simulink model "spacecraft_attitude_model"  (R2024b)
settings: Solver=ode4  StartTime=t0  StopTime=tf  FixedStep=0.1  RelTol=1e-3
values from neighbouring files (symbols this model uses):
  a = (((T/(2*pi))^2*mu_earth)^(1/3))    (= 7069867.85099)    [main_spacecraft_attitude_dynamics.m]
  A_body1 = surface(1)    [main_spacecraft_attitude_dynamics.m]
  A_body2 = surface(2)    [main_spacecraft_attitude_dynamics.m]
  A_body3 = surface(3)    [main_spacecraft_attitude_dynamics.m]
  A_body4 = surface(4)    [main_spacecraft_attitude_dynamics.m]
  A_body5 = surface(5)    [main_spacecraft_attitude_dynamics.m]
  A_body6 = surface(6)    [main_spacecraft_attitude_dynamics.m]
  A_panel1 = surface(7)    [main_spacecraft_attitude_dynamics.m]
  A_panel2 = surface(8)    [main_spacecraft_attitude_dynamics.m]
  A_panel3 = surface(9)    [main_spacecraft_attitude_dynamics.m]
  A_panel4 = surface(10)    [main_spacecraft_attitude_dynamics.m]
  alpha = [alpha1,alpha2,alpha3]    [main_spacecraft_attitude_dynamics.m]
  Ap = pinv(Ar)    [main_spacecraft_attitude_dynamics.m]
  Ar = Ar./norm(Ar)    [main_spacecraft_attitude_dynamics.m]
  AtmosphereModel = struct()    [AtmosphereData.m]    (also in main_spacecraft_attitude_dynamics.m)
  CD = 2.6    [main_spacecraft_attitude_dynamics.m]
  D_max = 50    [main_spacecraft_attitude_dynamics.m]
  Detumbling_time = 5000    [main_spacecraft_attitude_dynamics.m]
  e = 0.001    [main_spacecraft_attitude_dynamics.m]
  FOV = 128 * pi/180    (= 2.23402144255)    [main_spacecraft_attitude_dynamics.m]
  g1_0 = DGRF2020(1).g_nm    [main_spacecraft_attitude_dynamics.m]
  g1_1 = DGRF2020(2).g_nm    [main_spacecraft_attitude_dynamics.m]
  H = 700    [main_spacecraft_attitude_dynamics.m]
  h0 = 0    [main_spacecraft_attitude_dynamics.m]
  h1_1 = DGRF2020(2).h_nm    [main_spacecraft_attitude_dynamics.m]
  i = deg2rad(98.18)    [main_spacecraft_attitude_dynamics.m]
  Ir = 0.1    [main_spacecraft_attitude_dynamics.m]
  J = EXTRACTED_DATA.I_total    [main_spacecraft_attitude_dynamics.m]
  j_B = [0.01, 0.05, 0.01]'    [main_spacecraft_attitude_dynamics.m]
  k1 = max(max(kd_slew))    [main_spacecraft_attitude_dynamics.m]
  k2 = max(max(kp_slew))    [main_spacecraft_attitude_dynamics.m]
  Kw = max(max(kp_detumbling))    [main_spacecraft_attitude_dynamics.m]
  n = sqrt((G*M_E)/(r_earth^3))    [main_spacecraft_attitude_dynamics.m]
  N_B1 = N_B(1, :)'    [main_spacecraft_attitude_dynamics.m]
  N_B2 = N_B(2, :)'    [main_spacecraft_attitude_dynamics.m]
  N_B3 = N_B(3, :)'    [main_spacecraft_attitude_dynamics.m]
  N_B4 = N_B(4, :)'    [main_spacecraft_attitude_dynamics.m]
  N_B5 = N_B(5, :)'    [main_spacecraft_attitude_dynamics.m]
  N_B6 = N_B(6, :)'    [main_spacecraft_attitude_dynamics.m]
  N_P1 = N_B(7, :)'    [main_spacecraft_attitude_dynamics.m]
  N_P2 = N_B(8, :)'    [main_spacecraft_attitude_dynamics.m]
  N_P3 = N_B(9, :)'    [main_spacecraft_attitude_dynamics.m]
  N_P4 = N_B(10, :)'    [main_spacecraft_attitude_dynamics.m]
  n_S = (2*pi)/T_S    (= 1.99238499086e-07)    [main_spacecraft_attitude_dynamics.m]
  om = deg2rad(0)    [main_spacecraft_attitude_dynamics.m]
  P = Fe/c    (= 4.52980041279e-06)    [main_spacecraft_attitude_dynamics.m]
  pd_body1 = rho_D(1)    [main_spacecraft_attitude_dynamics.m]
  pd_body2 = rho_D(2)    [main_spacecraft_attitude_dynamics.m]
  pd_body3 = rho_D(3)    [main_spacecraft_attitude_dynamics.m]
  pd_body4 = rho_D(4)    [main_spacecraft_attitude_dynamics.m]
  pd_body5 = rho_D(5)    [main_spacecraft_attitude_dynamics.m]
  pd_body6 = rho_D(6)    [main_spacecraft_attitude_dynamics.m]
  pd_panel1 = rho_D(7)    [main_spacecraft_attitude_dynamics.m]
  pd_panel2 = rho_D(8)    [main_spacecraft_attitude_dynamics.m]
  pd_panel3 = rho_D(9)    [main_spacecraft_attitude_dynamics.m]
  pd_panel4 = rho_D(10)    [main_spacecraft_attitude_dynamics.m]
  ps_body1 = rho_S(1)    [main_spacecraft_attitude_dynamics.m]
  ps_body2 = rho_S(2)    [main_spacecraft_attitude_dynamics.m]
  ps_body3 = rho_S(3)    [main_spacecraft_attitude_dynamics.m]
  ps_body4 = rho_S(4)    [main_spacecraft_attitude_dynamics.m]
  ps_body5 = rho_S(5)    [main_spacecraft_attitude_dynamics.m]
  ps_body6 = rho_S(6)    [main_spacecraft_attitude_dynamics.m]
  ps_panel1 = rho_S(7)    [main_spacecraft_attitude_dynamics.m]
  ps_panel2 = rho_S(8)    [main_spacecraft_attitude_dynamics.m]
  ps_panel3 = rho_S(9)    [main_spacecraft_attitude_dynamics.m]
  ps_panel4 = rho_S(10)    [main_spacecraft_attitude_dynamics.m]
  q0 = [q1_0 q2_0 q3_0 q4_0]    [main_spacecraft_attitude_dynamics.m]
  r_earth = (R_earth + H)*10^3    (= 7078136.3)    [main_spacecraft_attitude_dynamics.m]
  R_earth = 6378.1363    [main_spacecraft_attitude_dynamics.m]
  r_f1 = r_F(1, :)'    [main_spacecraft_attitude_dynamics.m]
  r_f10 = r_F(10, :)'    [main_spacecraft_attitude_dynamics.m]
  r_f2 = r_F(2, :)'    [main_spacecraft_attitude_dynamics.m]
  r_f3 = r_F(3, :)'    [main_spacecraft_attitude_dynamics.m]
  r_f4 = r_F(4, :)'    [main_spacecraft_attitude_dynamics.m]
  r_f5 = r_F(5, :)'    [main_spacecraft_attitude_dynamics.m]
  r_f6 = r_F(6, :)'    [main_spacecraft_attitude_dynamics.m]
  r_f7 = r_F(7, :)'    [main_spacecraft_attitude_dynamics.m]
  r_f8 = r_F(8, :)'    [main_spacecraft_attitude_dynamics.m]
  r_f9 = r_F(9, :)'    [main_spacecraft_attitude_dynamics.m]
  r_Sun = 149597870    [main_spacecraft_attitude_dynamics.m]
  RAAN = deg2rad(RAAN)    [main_spacecraft_attitude_dynamics.m]
  sigma_b = RRW*(pi/180)*(1/3600)*(1/sqrt(Ts))    [main_spacecraft_attitude_dynamics.m]
  sigma_mag = 10^-6    (= 1e-06)    [main_spacecraft_attitude_dynamics.m]
  sigma_n = ARW*(pi/180)*(1/60)*(1/sqrt(Ts))    [main_spacecraft_attitude_dynamics.m]
  T_coil_max = 50 * 45*10^-6    (= 0.00225)    [main_spacecraft_attitude_dynamics.m]
  th0 = 0    [main_spacecraft_attitude_dynamics.m]
  v0 = [0 0 0]    [main_spacecraft_attitude_dynamics.m]
  variance_Ss = (a_sun)^2    (= 3.24)    [main_spacecraft_attitude_dynamics.m]
  w_0 = [-3, 3, 3]'    [main_spacecraft_attitude_dynamics.m]
  w_E = (2*pi)/(24*60*60)    (= 7.27220521664e-05)    [main_spacecraft_attitude_dynamics.m]
  w_LN = [0 0 0]'    [main_spacecraft_attitude_dynamics.m]
undefined symbols (not defined in the file or in its folder): A_Ss_orienation
libraries: matrix_library x38, slpidlib x2, aerolibutil x1, vrlib x1
(part 3 of 4)

== system spacecraft_attitude_model/Slew & Pointing/Slew and Pointing/Subsystem ==
  q_referance : Inport
  q_measured : Inport  Port=2
  Demux : Demux
  Gain : Gain  Gain=[0 0 0 -1; 0 0 1 0; 0 -1 0 0; 1 0 0 0];
  Gain1 : Gain  Gain=[0 1 0 0; -1 0 0 0; 0 0 0 -1; 0 0 1 0];
  Gain2 : Gain  Gain=[0 0 -1 0; 0 0 0 -1; 1 0 0 0; 0 1 0 0];
  Gain3 : Gain  Gain=[1 0 0 0; 0 1 0 0; 0 0 1 0; 0 0 0 1];
  MatrixMultiply : Product  Multiplication=Matrix(*)
  Sum : Sum  Inputs=++++
  q_error : Outport
  wires:
  q_referance/1 -> Demux/1
  Demux/1 -> Gain/1
  Demux/3 -> Gain1/1
  Demux/2 -> Gain2/1
  Demux/4 -> Gain3/1
  Gain/1 -> Sum/1
  Gain2/1 -> Sum/2
  Gain1/1 -> Sum/3
  Gain3/1 -> Sum/4
  Sum/1 -> MatrixMultiply/1
  q_measured/1 -> MatrixMultiply/2
  MatrixMultiply/1 -> q_error/1

== system spacecraft_attitude_model/Slew & Pointing/Slew and Pointing/Subsystem1 ==
  A_LN : Inport
  Clock : Clock
  Clock1 : Clock
  If : If  NumInputs=4  IfExpression=u1>0 & u1<1  ElseIfExpressions=u2>0 & u2<1, u3>0 & u3<1, u4>0 & u4<1  ShowElse=off
  If Action Subsystem : Subsystem  TreatAsAtomicUnit=on
  If Action Subsystem1 : Subsystem  TreatAsAtomicUnit=on
  If Action Subsystem2 : Subsystem  TreatAsAtomicUnit=on
  If Action Subsystem3 : Subsystem  TreatAsAtomicUnit=on
  If Action Subsystem4 : Subsystem  TreatAsAtomicUnit=on
  If Action Subsystem5 : Subsystem  TreatAsAtomicUnit=on
  If1 : If  IfExpression=u1==0
  Merge : Merge  Inputs=4
  Ortonormalization : Subsystem
  Scope : Scope
  Subsystem : Subsystem
  Subsystem1 : Subsystem
  Subsystem2 : Subsystem
  Subsystem3 : Subsystem
  Switch : Switch  Criteria=u2 ~= 0  SaturateOnIntegerOverflow=off  InputSameDT=off
  q : Outport
  wires:
  A_LN/1 -> Ortonormalization/1(A_LN)
  If/1 -> If Action Subsystem/Action
  If Action Subsystem/1(quaternion_4) -> Merge/1
  Merge/1 -> If Action Subsystem5/1(In1), If Action Subsystem1/1(In1)
  Subsystem/1(q4) -> If Action Subsystem/1(q4), If/1
  Subsystem1/1(q1) -> If Action Subsystem2/1(q1), If/2
  Subsystem2/1(q2) -> If/3, If Action Subsystem3/1(q2)
  Subsystem3/1(q3) -> If Action Subsystem4/1(q3), If/4
  If/2 -> If Action Subsystem2/Action
  If/3 -> If Action Subsystem3/Action
  If/4 -> If Action Subsystem4/Action
  If Action Subsystem2/1(quaternion_1) -> Merge/2
  If Action Subsystem3/1(quaternion_2) -> Merge/3
  If Action Subsystem4/1(quaternion_3) -> Merge/4
  Ortonormalization/1(Out1) -> If Action Subsystem3/2(A_BN), If Action Subsystem4/2("A_BN "), If Action Subsystem/2("A_BN "), If Action Subsystem2/2("A_BN "), Subsystem3/1(A_BN), Subsystem/1(A_BN), Subsystem1/1(A_BN), Subsystem2/1(A_BN)
  Clock/1 -> If1/1
  If1/1 -> If Action Subsystem1/Action
  If1/2 -> If Action Subsystem5/Action
  If Action Subsystem1/1(q) -> Switch/3
  If Action Subsystem5/1(q) -> Switch/1
  Switch/1 -> Scope/1, q/1
  Clock1/1 -> Switch/2

== system spacecraft_attitude_model/Slew & Pointing/Slew and Pointing/Subsystem2 ==
  q : Inport
  Clock : Clock
  Clock1 : Clock
  If Action Subsystem1 : Subsystem  TreatAsAtomicUnit=on
  If Action Subsystem5 : Subsystem  TreatAsAtomicUnit=on
  If1 : If  IfExpression=u1==0
  Scope1 : Scope
  Switch : Switch  Criteria=u2 ~= 0  SaturateOnIntegerOverflow=off  InputSameDT=off
  q_referance : Outport
  wires:
  If Action Subsystem1/1(q) -> Switch/3
  If Action Subsystem5/1(q_) -> Switch/1
  If1/1 -> If Action Subsystem1/Action
  Clock/1 -> If1/1
  Switch/1 -> q_referance/1, Scope1/1
  Clock1/1 -> Switch/2
  If1/2 -> If Action Subsystem5/Action
  q/1 -> If Action Subsystem1/1(Input), If Action Subsystem5/1(In1)

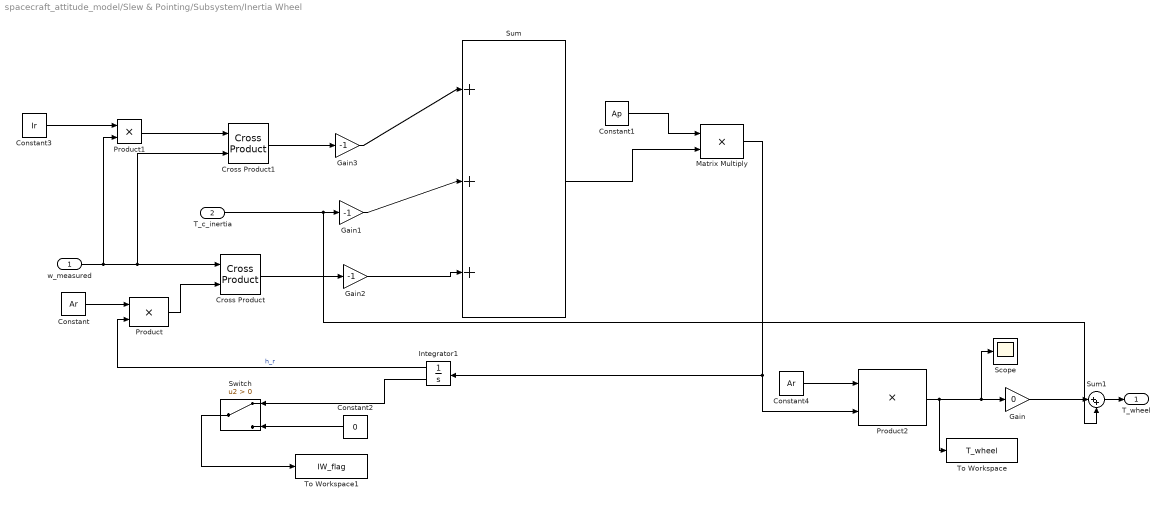
== system spacecraft_attitude_model/Slew & Pointing/Subsystem/Inertia Wheel ==
  w_measured : Inport
  T_c_inertia : Inport  Port=2
  Constant : Constant  Value=Ar
  Constant1 : Constant  Value=Ap
  Constant2 : Constant  Value=0
  Constant3 : Constant  Value=Ir
  Constant4 : Constant  Value=Ar
  Cross Product : matrix_library/Cross Product
  Cross Product1 : matrix_library/Cross Product
  Gain : Gain  Gain=0
  Gain1 : Gain  Gain=-1
  Gain2 : Gain  Gain=-1
  Gain3 : Gain  Gain=-1
  Integrator1 : Integrator  InitialCondition=h0  LimitOutput=on  UpperSaturationLimit=0.005  LowerSaturationLimit=-0.005  ShowSaturationPort=on
  Matrix Multiply : Product
  Product : Product
  Product1 : Product
  Product2 : Product
  Scope : Scope
  Sum : Sum  Inputs=|+++
  Sum1 : Sum  Inputs=|++
  Switch : Switch  Criteria=u2 > Threshold  SaturateOnIntegerOverflow=off  InputSameDT=off
  To Workspace : ToWorkspace  VariableName=T_wheel  SampleTime=-1
  To Workspace1 : ToWorkspace  VariableName=IW_flag  SampleTime=-1
  T_wheel : Outport
  wires:
  Product/1 -> Cross Product/2
  Cross Product/1 -> Gain2/1
  w_measured/1 -> Product1/2, Cross Product1/2, Cross Product/1
  Gain2/1 -> Sum/3
  Constant1/1 -> Matrix Multiply/1
  Gain3/1 -> Sum/1
  Matrix Multiply/1 -> Product2/2, Integrator1/1
  Constant3/1 -> Product1/1
  Integrator1/1 -> Product/2  "h_r"
  Integrator1/2 -> Switch/1
  Constant2/1 -> Switch/3
  Constant/1 -> Product/1
  Product2/1 -> To Workspace/1, Scope/1, Gain/1
  Gain1/1 -> Sum/2
  Switch/1 -> To Workspace1/1
  Product1/1 -> Cross Product1/1
  Cross Product1/1 -> Gain3/1
  Constant4/1 -> Product2/1
  T_c_inertia/1 -> Sum1/2, Gain1/1
  Sum/1 -> Matrix Multiply/2
  Gain/1 -> Sum1/1
  Sum1/1 -> T_wheel/1

== system spacecraft_attitude_model/Slew & Pointing/Subsystem/Magnetic coils ==
  T_Control : Inport
  b_measured : Inport  Port=2
  Demux : Demux  Outputs=3
  Demux1 : Demux  Outputs=3
  Gain : Gain
  Gain1 : Gain
  Gain2 : Gain
  Norm1 : Subsystem
      settings: PortSchema="{\"entries\":[{\"content\":{\"sides\":[{\"content\":{},\"type\":\"ConnectorPlacement.EquallySpacedRectSide\",\"uuid\":\"c8e6b557-1f56-4290-9ece-bfc368650609\"},{\"content\":{\"connectorIds\":[\"Out1\"],\"side\":\"RIGHT\"},\"type\":\"ConnectorPlacement.EquallySpacedRectSide\",\"uuid\":\"77fa52b5-00ea-4466-8814-b89029d0f61f\"},{\"content\":{\"connectorIds\":[\"In1\"],\"side\":\"TOP\"},\"type\":\"ConnectorPlacement.EquallySpacedRectSide\",\"uuid\":\"5a1e965d-5eef-4834-963c-decfdd4da2be\"},{\"content\":{\"side\":\"BOTTOM\"},\"type\":\"ConnectorPlacement.EquallySpacedRectSide\",\"uuid\":\"d0b05173-3d81-4b7c-baba-8d47e4810e0f\"}]},\"type\":\"ConnectorPlacement.EquallySpacedConnector\",\"uuid\":\"bc13670f-664f-40fc-b4f3-9fab538d09d1\"}],\"packageUris\":[\"http://schema.mathworks.com/mf0/Connector/R2020b\"],\"version\":\"1.0\"}"
  Scope2 : Scope
  Square1 : Math  Operator=square
  Subsystem : Subsystem
  Subsystem1 : Subsystem
  Subsystem2 : Subsystem
  Vector Concatenate : Concatenate  NumInputs=3
  T_coils : Outport
  wires:
  Square1/1 -> Subsystem/3(b_norm^2), Subsystem1/3(b_norm^2), Subsystem2/3(b_norm^2)
  Demux1/2 -> Subsystem1/2(b_y)
  Demux/1 -> Gain/1
  Demux1/1 -> Subsystem/2(b_x)
  Gain1/1 -> Subsystem1/1(T_y)
  Gain/1 -> Subsystem/1(T_x)
  Gain2/1 -> Subsystem2/1(T_z)
  Demux1/3 -> Subsystem2/2(b_z)
  Demux/3 -> Gain2/1
  b_measured/1 -> Norm1/1(b), Demux1/1
  Norm1/1(b_norm) -> Square1/1  "b_norm"
  Demux/2 -> Gain1/1
  Vector Concatenate/1 -> T_coils/1, Scope2/1
  T_Control/1 -> Demux/1
  Subsystem2/1(T_coil_z) -> Vector Concatenate/3
  Subsystem1/1(T_coil_y) -> Vector Concatenate/2
  Subsystem/1(T_coil_x) -> Vector Concatenate/1

== system spacecraft_attitude_model/Sun Sensor /Alpha Beta1/Subsystem ==
  In1 : Inport
  Atan1 : Trigonometry  Operator=atan2
  Atan2 : Trigonometry  Operator=atan2
  Demux : Demux  Outputs=3
  Out1 : Outport
  Out2 : Outport  Port=2
  wires:
  Demux/3 -> Atan2/2, Atan1/2  "Sz"
  Atan1/1 -> Out2/1
  Demux/1 -> Atan2/1  "Sx"
  In1/1 -> Demux/1
  Demux/2 -> Atan1/1  "Sy"
  Atan2/1 -> Out1/1

== system spacecraft_attitude_model/Sun Sensor /Alpha Beta1/Subsystem1 ==
  In1 : Inport
  Atan1 : Trigonometry  Operator=atan2
  Atan2 : Trigonometry  Operator=atan2
  Demux : Demux  Outputs=3
  Out1 : Outport
  Out2 : Outport  Port=2
  wires:
  Demux/3 -> Atan2/2, Atan1/2  "Sz"
  Atan1/1 -> Out2/1
  Demux/1 -> Atan2/1  "Sx"
  In1/1 -> Demux/1
  Demux/2 -> Atan1/1  "Sy"
  Atan2/1 -> Out1/1

== system spacecraft_attitude_model/Sun Sensor /Alpha Beta1/Subsystem2 ==
  In1 : Inport
  Atan1 : Trigonometry  Operator=atan2
  Atan2 : Trigonometry  Operator=atan2
  Demux : Demux  Outputs=3
  Out1 : Outport
  Out2 : Outport  Port=2
  wires:
  Demux/3 -> Atan2/2, Atan1/2  "Sz"
  Atan1/1 -> Out2/1
  Demux/1 -> Atan2/1  "Sx"
  In1/1 -> Demux/1
  Demux/2 -> Atan1/1  "Sy"
  Atan2/1 -> Out1/1

== system spacecraft_attitude_model/Sun Sensor /Alpha Beta1/Subsystem3 ==
  In1 : Inport
  Atan1 : Trigonometry  Operator=atan2
  Atan2 : Trigonometry  Operator=atan2
  Demux : Demux  Outputs=3
  Out1 : Outport
  Out2 : Outport  Port=2
  wires:
  Demux/3 -> Atan2/2, Atan1/2  "Sz"
  Atan1/1 -> Out2/1
  Demux/1 -> Atan2/1  "Sx"
  In1/1 -> Demux/1
  Demux/2 -> Atan1/1  "Sy"
  Atan2/1 -> Out1/1

== system spacecraft_attitude_model/Sun Sensor /Alpha Beta1/Subsystem4 ==
  In1 : Inport
  Atan1 : Trigonometry  Operator=atan2
  Atan2 : Trigonometry  Operator=atan2
  Demux : Demux  Outputs=3
  Out1 : Outport
  Out2 : Outport  Port=2
  wires:
  Demux/3 -> Atan2/2, Atan1/2  "Sz"
  Atan1/1 -> Out2/1
  Demux/1 -> Atan2/1  "Sx"
  In1/1 -> Demux/1
  Demux/2 -> Atan1/1  "Sy"
  Atan2/1 -> Out1/1

== system spacecraft_attitude_model/Sun Sensor /Alpha Beta1/Subsystem5 ==
  In1 : Inport
  Atan1 : Trigonometry  Operator=atan2
  Atan2 : Trigonometry  Operator=atan2
  Demux : Demux  Outputs=3
  Out1 : Outport
  Out2 : Outport  Port=2
  wires:
  Demux/3 -> Atan2/2, Atan1/2  "Sz"
  Atan1/1 -> Out2/1
  Demux/1 -> Atan2/1  "Sx"
  In1/1 -> Demux/1
  Demux/2 -> Atan1/1  "Sy"
  Atan2/1 -> Out1/1

== system spacecraft_attitude_model/Detumbling/Subsystem4/Magnetic coils/Norm1 ==
  b : Inport
  Demux : Demux  Outputs=3
  Sqrt : Sqrt
  Square : Math  Operator=square
  Square1 : Math  Operator=square
  Square2 : Math  Operator=square
  Sum : Sum  Inputs=|+++
  b_norm : Outport
  wires:
  Demux/3 -> Square2/1
  b/1 -> Demux/1
  Demux/1 -> Square/1
  Demux/2 -> Square1/1
  Square/1 -> Sum/1
  Square1/1 -> Sum/2
  Square2/1 -> Sum/3
  Sum/1 -> Sqrt/1
  Sqrt/1 -> b_norm/1

== system spacecraft_attitude_model/Detumbling/Subsystem4/Magnetic coils/Subsystem ==
  T_x : Inport
  b_x : Inport  Port=2
  b_norm^2 : Inport  Port=3
  Divide2 : Product  Inputs=*/
  Product : Product
  Product1 : Product
  Saturation2 : Saturate  UpperLimit=T_coil_max  LowerLimit=-T_coil_max
  Saturation3 : Saturate  UpperLimit=D_max  LowerLimit=-D_max
  Scope2 : Scope
  Scope3 : Scope
  T_coil_x : Outport
  wires:
  Saturation3/1 -> Product1/1
  Divide2/1 -> Scope3/1, Saturation3/1
  Product/1 -> Divide2/1
  Product1/1 -> Saturation2/1  "T_coils_x"
  b_norm^2/1 -> Divide2/2
  b_x/1 -> Product1/2, Product/2
  T_x/1 -> Product/1
  Saturation2/1 -> Scope2/1, T_coil_x/1

== system spacecraft_attitude_model/Detumbling/Subsystem4/Magnetic coils/Subsystem1 ==
  T_y : Inport
  b_y : Inport  Port=2
  b_norm^2 : Inport  Port=3
  Divide2 : Product  Inputs=*/
  Product : Product
  Product1 : Product
  Saturation2 : Saturate  UpperLimit=T_coil_max  LowerLimit=-T_coil_max
  Saturation3 : Saturate  UpperLimit=D_max  LowerLimit=-D_max
  Scope2 : Scope
  Scope3 : Scope
  T_coil_y : Outport
  wires:
  Saturation3/1 -> Product1/1
  Divide2/1 -> Scope3/1, Saturation3/1
  Product/1 -> Divide2/1
  Product1/1 -> Saturation2/1
  b_norm^2/1 -> Divide2/2
  b_y/1 -> Product1/2, Product/2
  T_y/1 -> Product/1
  Saturation2/1 -> Scope2/1, T_coil_y/1

== system spacecraft_attitude_model/Detumbling/Subsystem4/Magnetic coils/Subsystem2 ==
  T_z : Inport
  b_z : Inport  Port=2
  b_norm^2 : Inport  Port=3
  Divide2 : Product  Inputs=*/
  Product : Product
  Product1 : Product
  Saturation2 : Saturate  UpperLimit=T_coil_max  LowerLimit=-T_coil_max
  Saturation3 : Saturate  UpperLimit=D_max  LowerLimit=-D_max
  Scope2 : Scope
  Scope3 : Scope
  T_coil_z : Outport
  wires:
  Saturation3/1 -> Product1/1
  Divide2/1 -> Scope3/1, Saturation3/1
  Product/1 -> Divide2/1
  Product1/1 -> Saturation2/1
  b_norm^2/1 -> Divide2/2
  b_z/1 -> Product1/2, Product/2
  T_z/1 -> Product/1
  Saturation2/1 -> Scope2/1, T_coil_z/1

== system spacecraft_attitude_model/Disturbances Torque/Air Drag/A_Cross/A_CROSS1 ==
  v_r_hat : Inport
  A_1 : Constant  Value=A_body1
  Constant : Constant  Value=0
  Dot Product : DotProduct  OutDataTypeStr=Inherit: Inherit via internal rule
  Product : Product
  Switch : Switch  SaturateOnIntegerOverflow=off  InputSameDT=off
  n_s1 : Constant  Value=N_B1
  A_cross1 : Outport
  wires:
  n_s1/1 -> Dot Product/1
  Dot Product/1 -> Product/2, Switch/2
  Switch/1 -> A_cross1/1
  Constant/1 -> Switch/3
  Product/1 -> Switch/1
  A_1/1 -> Product/1
  v_r_hat/1 -> Dot Product/2

== system spacecraft_attitude_model/Disturbances Torque/Air Drag/A_Cross/A_CROSS10 ==
  v_r_hat : Inport
  A_10 : Constant  Value=A_panel4
  Constant : Constant  Value=0
  Dot Product : DotProduct  OutDataTypeStr=Inherit: Inherit via internal rule
  Product : Product
  Switch : Switch  SaturateOnIntegerOverflow=off  InputSameDT=off
  n_s10 : Constant  Value=N_P4
  A_cross10 : Outport
  wires:
  n_s10/1 -> Dot Product/1
  Dot Product/1 -> Product/2, Switch/2
  Switch/1 -> A_cross10/1
  Constant/1 -> Switch/3
  Product/1 -> Switch/1
  A_10/1 -> Product/1
  v_r_hat/1 -> Dot Product/2

== system spacecraft_attitude_model/Disturbances Torque/Air Drag/A_Cross/A_CROSS2 ==
  v_r_hat : Inport
  A_2 : Constant  Value=A_body2
  Constant : Constant  Value=0
  Dot Product : DotProduct  OutDataTypeStr=Inherit: Inherit via internal rule
  Product : Product
  Switch : Switch  SaturateOnIntegerOverflow=off  InputSameDT=off
  n_s2 : Constant  Value=N_B2
  A_cross2 : Outport
  wires:
  n_s2/1 -> Dot Product/1
  Dot Product/1 -> Product/2, Switch/2
  Switch/1 -> A_cross2/1
  Constant/1 -> Switch/3
  Product/1 -> Switch/1
  A_2/1 -> Product/1
  v_r_hat/1 -> Dot Product/2

== system spacecraft_attitude_model/Disturbances Torque/Air Drag/A_Cross/A_CROSS3 ==
  v_r_hat : Inport
  A_3 : Constant  Value=A_body3
  Constant : Constant  Value=0
  Dot Product : DotProduct  OutDataTypeStr=Inherit: Inherit via internal rule
  Product : Product
  Switch : Switch  SaturateOnIntegerOverflow=off  InputSameDT=off
  n_s3 : Constant  Value=N_B3
  A_cross3 : Outport
  wires:
  n_s3/1 -> Dot Product/1
  Dot Product/1 -> Product/2, Switch/2
  Switch/1 -> A_cross3/1
  Constant/1 -> Switch/3
  Product/1 -> Switch/1
  A_3/1 -> Product/1
  v_r_hat/1 -> Dot Product/2

== system spacecraft_attitude_model/Disturbances Torque/Air Drag/A_Cross/A_CROSS4 ==
  v_r_hat : Inport
  A_4 : Constant  Value=A_body4
  Constant : Constant  Value=0
  Dot Product : DotProduct  OutDataTypeStr=Inherit: Inherit via internal rule
  Product : Product
  Switch : Switch  SaturateOnIntegerOverflow=off  InputSameDT=off
  n_s4 : Constant  Value=N_B4
  A_cross4 : Outport
  wires:
  n_s4/1 -> Dot Product/1
  Dot Product/1 -> Product/2, Switch/2
  Switch/1 -> A_cross4/1
  Constant/1 -> Switch/3
  Product/1 -> Switch/1
  A_4/1 -> Product/1
  v_r_hat/1 -> Dot Product/2

== system spacecraft_attitude_model/Disturbances Torque/Air Drag/A_Cross/A_CROSS5 ==
  v_r_hat : Inport
  A_5 : Constant  Value=A_body5
  Constant : Constant  Value=0
  Dot Product : DotProduct  OutDataTypeStr=Inherit: Inherit via internal rule
  Product : Product
  Switch : Switch  SaturateOnIntegerOverflow=off  InputSameDT=off
  n_s5 : Constant  Value=N_B5
  A_cross2 : Outport
  wires:
  n_s5/1 -> Dot Product/1
  Dot Product/1 -> Product/2, Switch/2
  Switch/1 -> A_cross2/1
  Constant/1 -> Switch/3
  Product/1 -> Switch/1
  A_5/1 -> Product/1
  v_r_hat/1 -> Dot Product/2

== system spacecraft_attitude_model/Disturbances Torque/Air Drag/A_Cross/A_CROSS6 ==
  v_r_hat : Inport
  A_6 : Constant  Value=A_body6
  Constant : Constant  Value=0
  Dot Product : DotProduct  OutDataTypeStr=Inherit: Inherit via internal rule
  Product : Product
  Switch : Switch  SaturateOnIntegerOverflow=off  InputSameDT=off
  n_s6 : Constant  Value=N_B6
  A_cross6 : Outport
  wires:
  n_s6/1 -> Dot Product/1
  Dot Product/1 -> Product/2, Switch/2
  Switch/1 -> A_cross6/1
  Constant/1 -> Switch/3
  Product/1 -> Switch/1
  A_6/1 -> Product/1
  v_r_hat/1 -> Dot Product/2

== system spacecraft_attitude_model/Disturbances Torque/Air Drag/A_Cross/A_CROSS7 ==
  v_r_hat : Inport
  A_7 : Constant  Value=A_panel1
  Constant : Constant  Value=0
  Dot Product : DotProduct  OutDataTypeStr=Inherit: Inherit via internal rule
  Product : Product
  Switch : Switch  SaturateOnIntegerOverflow=off  InputSameDT=off
  n_s7 : Constant  Value=N_P1
  A_cross7 : Outport
  wires:
  n_s7/1 -> Dot Product/1
  Dot Product/1 -> Product/2, Switch/2
  Switch/1 -> A_cross7/1
  Constant/1 -> Switch/3
  Product/1 -> Switch/1
  A_7/1 -> Product/1
  v_r_hat/1 -> Dot Product/2

== system spacecraft_attitude_model/Disturbances Torque/Air Drag/A_Cross/A_CROSS8 ==
  v_r_hat : Inport
  A_8 : Constant  Value=A_panel2
  Constant : Constant  Value=0
  Dot Product : DotProduct  OutDataTypeStr=Inherit: Inherit via internal rule
  Product : Product
  Switch : Switch  SaturateOnIntegerOverflow=off  InputSameDT=off
  n_s8 : Constant  Value=N_P2
  A_cross8 : Outport
  wires:
  n_s8/1 -> Dot Product/1
  Dot Product/1 -> Product/2, Switch/2
  Switch/1 -> A_cross8/1
  Constant/1 -> Switch/3
  Product/1 -> Switch/1
  A_8/1 -> Product/1
  v_r_hat/1 -> Dot Product/2

== system spacecraft_attitude_model/Disturbances Torque/Air Drag/A_Cross/A_CROSS9 ==
  v_r_hat : Inport
  A_9 : Constant  Value=A_panel3
  Constant : Constant  Value=0
  Dot Product : DotProduct  OutDataTypeStr=Inherit: Inherit via internal rule
  Product : Product
  Switch : Switch  SaturateOnIntegerOverflow=off  InputSameDT=off
  n_s9 : Constant  Value=N_P3
  A_cross9 : Outport
  wires:
  n_s9/1 -> Dot Product/1
  Dot Product/1 -> Product/2, Switch/2
  Switch/1 -> A_cross9/1
  Constant/1 -> Switch/3
  Product/1 -> Switch/1
  A_9/1 -> Product/1
  v_r_hat/1 -> Dot Product/2

== system spacecraft_attitude_model/Disturbances Torque/Air Drag/Subsystem1/F1 ==
  v_rB^2 : Inport
  v_rB_hat : Inport  Port=2
  A_cross1 : Inport  Port=3
  Constant : Constant  Value=-1/2
  Constant1 : Constant  Value=CD
  Product : Product  Inputs=6
  rho : Constant  Value=AtmosphereModel(H/100).Density_kg_m3/10^6
  Out1 : Outport
  wires:
  rho/1 -> Product/2
  Constant1/1 -> Product/3
  Constant/1 -> Product/1
  v_rB^2/1 -> Product/4
  Product/1 -> Out1/1
  v_rB_hat/1 -> Product/5
  A_cross1/1 -> Product/6

== system spacecraft_attitude_model/Disturbances Torque/Air Drag/Subsystem1/F10 ==
  v_rB^2 : Inport
  v_rB_hat : Inport  Port=2
  A_cross10 : Inport  Port=3
  Constant : Constant  Value=-1/2
  Constant1 : Constant  Value=CD
  Product : Product  Inputs=6
  rho : Constant  Value=AtmosphereModel(H/100).Density_kg_m3/10^6
  Out1 : Outport
  wires:
  rho/1 -> Product/2
  Constant1/1 -> Product/3
  Constant/1 -> Product/1
  v_rB^2/1 -> Product/4
  Product/1 -> Out1/1
  v_rB_hat/1 -> Product/5
  A_cross10/1 -> Product/6

== system spacecraft_attitude_model/Disturbances Torque/Air Drag/Subsystem1/F2 ==
  v_rB^2 : Inport
  v_rB_hat : Inport  Port=2
  A_cross2 : Inport  Port=3
  Constant : Constant  Value=-1/2
  Constant1 : Constant  Value=CD
  Product : Product  Inputs=6
  rho : Constant  Value=AtmosphereModel(H/100).Density_kg_m3/10^6
  Out1 : Outport
  wires:
  rho/1 -> Product/2
  Constant1/1 -> Product/3
  Constant/1 -> Product/1
  v_rB^2/1 -> Product/4
  Product/1 -> Out1/1
  v_rB_hat/1 -> Product/5
  A_cross2/1 -> Product/6

== system spacecraft_attitude_model/Disturbances Torque/Air Drag/Subsystem1/F3 ==
  v_rB^2 : Inport
  v_rB_hat : Inport  Port=2
  A_cross3 : Inport  Port=3
  Constant : Constant  Value=-1/2
  Constant1 : Constant  Value=CD
  Product : Product  Inputs=6
  rho : Constant  Value=AtmosphereModel(H/100).Density_kg_m3/10^6
  Out1 : Outport
  wires:
  rho/1 -> Product/2
  Constant1/1 -> Product/3
  Constant/1 -> Product/1
  v_rB^2/1 -> Product/4
  Product/1 -> Out1/1
  v_rB_hat/1 -> Product/5
  A_cross3/1 -> Product/6

== system spacecraft_attitude_model/Disturbances Torque/Air Drag/Subsystem1/F4 ==
  v_rB^2 : Inport
  v_rB_hat : Inport  Port=2
  A_cross4 : Inport  Port=3
  Constant : Constant  Value=-1/2
  Constant1 : Constant  Value=CD
  Product : Product  Inputs=6
  rho : Constant  Value=AtmosphereModel(H/100).Density_kg_m3/10^6
  Out1 : Outport
  wires:
  rho/1 -> Product/2
  Constant1/1 -> Product/3
  Constant/1 -> Product/1
  v_rB^2/1 -> Product/4
  Product/1 -> Out1/1
  v_rB_hat/1 -> Product/5
  A_cross4/1 -> Product/6

== system spacecraft_attitude_model/Disturbances Torque/Air Drag/Subsystem1/F5 ==
  v_rB^2 : Inport
  v_rB_hat : Inport  Port=2
  A_cross5 : Inport  Port=3
  Constant : Constant  Value=-1/2
  Constant1 : Constant  Value=CD
  Product : Product  Inputs=6
  rho : Constant  Value=AtmosphereModel(H/100).Density_kg_m3/10^6
  Out1 : Outport
  wires:
  rho/1 -> Product/2
  Constant1/1 -> Product/3
  Constant/1 -> Product/1
  v_rB^2/1 -> Product/4
  Product/1 -> Out1/1
  v_rB_hat/1 -> Product/5
  A_cross5/1 -> Product/6

== system spacecraft_attitude_model/Disturbances Torque/Air Drag/Subsystem1/F6 ==
  v_rB^2 : Inport
  v_rB_hat : Inport  Port=2
  A_cross6 : Inport  Port=3
  Constant : Constant  Value=-1/2
  Constant1 : Constant  Value=CD
  Product : Product  Inputs=6
  rho : Constant  Value=AtmosphereModel(H/100).Density_kg_m3/10^6
  Out1 : Outport
  wires:
  rho/1 -> Product/2
  Constant1/1 -> Product/3
  Constant/1 -> Product/1
  v_rB^2/1 -> Product/4
  Product/1 -> Out1/1
  v_rB_hat/1 -> Product/5
  A_cross6/1 -> Product/6

== system spacecraft_attitude_model/Disturbances Torque/Air Drag/Subsystem1/F7 ==
  v_rB^2 : Inport
  v_rB_hat : Inport  Port=2
  A_cross7 : Inport  Port=3
  Constant : Constant  Value=-1/2
  Constant1 : Constant  Value=CD
  Product : Product  Inputs=6
  rho : Constant  Value=AtmosphereModel(H/100).Density_kg_m3/10^6
  Out1 : Outport
  wires:
  rho/1 -> Product/2
  Constant1/1 -> Product/3
  Constant/1 -> Product/1
  v_rB^2/1 -> Product/4
  Product/1 -> Out1/1
  v_rB_hat/1 -> Product/5
  A_cross7/1 -> Product/6

== system spacecraft_attitude_model/Disturbances Torque/Air Drag/Subsystem1/F8 ==
  v_rB^2 : Inport
  v_rB_hat : Inport  Port=2
  A_cross8 : Inport  Port=3
  Constant : Constant  Value=-1/2
  Constant1 : Constant  Value=CD
  Product : Product  Inputs=6
  rho : Constant  Value=AtmosphereModel(H/100).Density_kg_m3/10^6
  Out1 : Outport
  wires:
  rho/1 -> Product/2
  Constant1/1 -> Product/3
  Constant/1 -> Product/1
  v_rB^2/1 -> Product/4
  Product/1 -> Out1/1
  v_rB_hat/1 -> Product/5
  A_cross8/1 -> Product/6

== system spacecraft_attitude_model/Disturbances Torque/Air Drag/Subsystem1/F9 ==
  v_rB^2 : Inport
  v_rB_hat : Inport  Port=2
  A_cross9 : Inport  Port=3
  Constant : Constant  Value=-1/2
  Constant1 : Constant  Value=CD
  Product : Product  Inputs=6
  rho : Constant  Value=AtmosphereModel(H/100).Density_kg_m3/10^6
  Out1 : Outport
  wires:
  rho/1 -> Product/2
  Constant1/1 -> Product/3
  Constant/1 -> Product/1
  v_rB^2/1 -> Product/4
  Product/1 -> Out1/1
  v_rB_hat/1 -> Product/5
  A_cross9/1 -> Product/6

== system spacecraft_attitude_model/Disturbances Torque/Gravity Gradient/Gravity Gradient/c ==
  A_BL : Inport
  Constant : Constant  Value=0
  Constant1 : Constant
  Matrix Multiply : Product  Multiplication=Matrix(*)
  Mux : Mux  Inputs=3
  c : Outport
  wires:
  Constant1/1 -> Mux/1
  Constant/1 -> Mux/3, Mux/2
  A_BL/1 -> Matrix Multiply/1
  Mux/1 -> Matrix Multiply/2
  Matrix Multiply/1 -> c/1

== system spacecraft_attitude_model/Envoirment/Model/Magnetic Field/H0 ==
  Constant : Constant  Value=(g1_0)^2
  Constant1 : Constant  Value=(g1_1)^2
  Constant2 : Constant  Value=(h1_1)^2
  Scope : Scope
  Sqrt : Sqrt
  Sum : Sum  Inputs=|+++
  To Workspace : ToWorkspace  VariableName=H0  SampleTime=-1
  H_0 : Outport
  wires:
  Constant2/1 -> Sum/3
  Sum/1 -> Sqrt/1
  Sqrt/1 -> To Workspace/1, Scope/1, H_0/1
  Constant/1 -> Sum/1
  Constant1/1 -> Sum/2

== system spacecraft_attitude_model/Envoirment/Model/Magnetic Field/b_Ned ==
  m : Inport
  H_0 : Inport  Port=2
  r_N : Inport  Port=3
  Constant : Constant  Value=3
  Constant1 : Constant  Value=(r_earth)^3
  Divide : Product  Inputs=*/
  Divide1 : Product  Inputs=*/
  Dot Product : DotProduct  OutDataTypeStr=Inherit: Inherit via internal rule
  Gain : Gain  Gain=3
  Norm : Subsystem
  Power : Math  Operator=pow
  Product : Product
  Product2 : Product
  Product3 : Product
  Scope : Scope
  Scope1 : Scope
  Scope2 : Scope
  Sum : Sum  Inputs=|+-
  b_N : Outport
  wires:
  H_0/1 -> Product/1
  m/1 -> Dot Product/1, Sum/2
  Dot Product/1 -> Product2/1  "m * r"
  r_N/1 -> Divide1/1, Norm/1(In1)
  Norm/1(Out1) -> Scope1/1, Power/1, Divide1/2  "r_norm"
  Divide1/1 -> Scope2/1, Dot Product/2, Product2/2  "r_versor"
  Constant/1 -> Power/2
  Product/1 -> Product3/2
  Product3/1 -> Divide/1
  Power/1 -> Divide/2
  Divide/1 -> Scope/1, b_N/1
  Sum/1 -> Product3/1  "3(m*r)r - m"
  Product2/1 -> Gain/1  "(m*r)r"
  Gain/1 -> Sum/1
  Constant1/1 -> Product/2

== system spacecraft_attitude_model/Envoirment/Model/Magnetic Field/m ==
  11.5 deg : Constant  Value=deg2rad(11.5)
  Clock : Clock
  Constant : Constant  Value=w_E
  Cos : Trigonometry  Operator=cos
  Cos1 : Trigonometry  Operator=cos
  Product : Product
  Product1 : Product
  Product2 : Product
  Scope : Scope
  Sin : Trigonometry
  Sin1 : Trigonometry
  Vector Concatenate : Concatenate  NumInputs=3
  m : Outport
  wires:
  Product2/1 -> Vector Concatenate/2
  Clock/1 -> Product/1
  11.5 deg/1 -> Sin/1, Cos/1
  Sin/1 -> Product2/1, Product1/1
  Cos1/1 -> Product1/2
  Cos/1 -> Vector Concatenate/3
  Sin1/1 -> Product2/2
  Constant/1 -> Product/2
  Product1/1 -> Vector Concatenate/1
  Vector Concatenate/1 -> Scope/1, m/1
  Product/1 -> Sin1/1, Cos1/1

== system spacecraft_attitude_model/Envoirment/Two_Body_Keplerian_Dynamics/Subsystem/rN ==
  r : Inport
  Theta : Inport  Port=2
  Constant : Constant  Value=deg2rad(98.18)
  Cos1 : Trigonometry  Operator=cos
  Cos3 : Trigonometry  Operator=cos
  Product{,1..4} (5 alike) : Product
  Sin : Trigonometry
  Sin1 : Trigonometry
  Vector Concatenate : Concatenate  NumInputs=3
  r_N : Outport
  wires:
  Theta/1 -> Cos3/1, Sin1/1
  Constant/1 -> Sin/1, Cos1/1
  Product4/1 -> Vector Concatenate/3  "r*sin(th)*sin(i)"
  Product/1 -> Vector Concatenate/1  "r*cos(th)"
  Product2/1 -> Vector Concatenate/2  "r*sin(th)*cos(i)"
  r/1 -> Product4/1, Product2/1, Product/1  "r"
  Sin1/1 -> Product3/1, Product1/1
  Product1/1 -> Product2/2
  Cos3/1 -> Product/2
  Sin/1 -> Product3/2
  Product3/1 -> Product4/2
  Vector Concatenate/1 -> r_N/1
  Cos1/1 -> Product1/2

== system spacecraft_attitude_model/Kinematics/quaternions to DCM/q2A_DCM/Creation of q vector skew Matrix ==
  q : Inport
  Constant : Constant  Value=[1 0 0]
  Constant1 : Constant  Value=[0 1 0]  VectorParams1D=off
  Constant2 : Constant  Value=[0 0 1]  VectorParams1D=off
  Cross Product : matrix_library/Cross Product
  Cross Product1 : matrix_library/Cross Product
  Cross Product2 : matrix_library/Cross Product
  Matrix Concatenate : Concatenate  NumInputs=3  Mode=Multidimensional array
  To Workspace1 : ToWorkspace  VariableName=q_skew  SampleTime=-1
  Transpose : matrix_library/Transpose
  "[q]^" : Outport
  wires:
  q/1 -> Cross Product/1, Cross Product1/1, Cross Product2/1
  Constant2/1 -> Cross Product2/2
  Cross Product1/1 -> Matrix Concatenate/2  "Line 2"
  Cross Product2/1 -> Matrix Concatenate/3  "Line 3"
  Cross Product/1 -> Matrix Concatenate/1  "Line 1"
  Matrix Concatenate/1 -> Transpose/1  "skew"
  Constant1/1 -> Cross Product1/2
  Constant/1 -> Cross Product/2
  Transpose/1 -> To Workspace1/1, "[q]^"/1

== system spacecraft_attitude_model/Slew & Pointing/Slew and Pointing/Subsystem1/If Action Subsystem ==
  q4 : Inport
  "A_BN " : Inport  Port=2
  Action Port : ActionPort  ActionPortLabel=if(u1>0 & u1<1)
  Divide : Product  Inputs=*/
  Divide1 : Product  Inputs=*/
  Divide2 : Product  Inputs=*/
  Gain1 : Gain  Gain=1/4
  Gain2 : Gain  Gain=1/4
  Gain3 : Gain  Gain=1/4
  Mux : Mux
  Selector : Selector  NumberOfDimensions=2  InputPortWidth=3  IndexOptions=Index vector (dialog),Index vector (dialog)  Indices=2,3  OutputSizes=1,1
  Selector1 : Selector  NumberOfDimensions=2  InputPortWidth=3  IndexOptions=Index vector (dialog),Index vector (dialog)  Indices=3,2  OutputSizes=1,1
  Selector2 : Selector  NumberOfDimensions=2  InputPortWidth=3  IndexOptions=Index vector (dialog),Index vector (dialog)  Indices=3,1  OutputSizes=1,1
  Selector3 : Selector  NumberOfDimensions=2  InputPortWidth=3  IndexOptions=Index vector (dialog),Index vector (dialog)  Indices=1,3  OutputSizes=1,1
  Selector4 : Selector  NumberOfDimensions=2  InputPortWidth=3  IndexOptions=Index vector (dialog),Index vector (dialog)  Indices=1,2  OutputSizes=1,1
  Selector6 : Selector  NumberOfDimensions=2  InputPortWidth=3  IndexOptions=Index vector (dialog),Index vector (dialog)  Indices=2,1  OutputSizes=1,1
  Sum1 : Sum  Inputs=+-
  Sum2 : Sum  Inputs=+-
  Sum3 : Sum  Inputs=+-
  quaternion_4 : Outport
  wires:
  Selector6/1 -> Sum3/2  "A21"
  Divide2/1 -> Mux/3  "q3"
  Sum3/1 -> Gain3/1
  Selector4/1 -> Sum3/1  "A12"
  Sum2/1 -> Gain2/1
  Gain3/1 -> Divide2/1
  Divide1/1 -> Mux/2  "q2"
  Divide/1 -> Mux/1  "q1"
  Selector3/1 -> Sum2/2  "A13"
  Selector/1 -> Sum1/1  "A23"
  Selector2/1 -> Sum2/1  "A31"
  Selector1/1 -> Sum1/2  "A32"
  Gain2/1 -> Divide1/1
  Sum1/1 -> Gain1/1
  Gain1/1 -> Divide/1
  q4/1 -> Mux/4, Divide2/2, Divide1/2, Divide/2
  "A_BN "/1 -> Selector6/1, Selector4/1, Selector3/1, Selector/1, Selector1/1, Selector2/1
  Mux/1 -> quaternion_4/1

== system spacecraft_attitude_model/Slew & Pointing/Slew and Pointing/Subsystem1/If Action Subsystem1 ==
  In1 : Inport
  Action Port : ActionPort  ActionPortLabel=if(u1==0)
  q : Outport
  wires:
  In1/1 -> q/1

== system spacecraft_attitude_model/Slew & Pointing/Slew and Pointing/Subsystem1/If Action Subsystem2 ==
  q1 : Inport
  "A_BN " : Inport  Port=2
  Action Port : ActionPort  ActionPortLabel=elseif(u2>0 & u2<1)
  Divide : Product  Inputs=*/
  Divide1 : Product  Inputs=*/
  Divide2 : Product  Inputs=*/
  Gain1 : Gain  Gain=1/4
  Gain2 : Gain  Gain=1/4
  Gain3 : Gain  Gain=1/4
  Mux : Mux
  Selector : Selector  NumberOfDimensions=2  InputPortWidth=3  IndexOptions=Index vector (dialog),Index vector (dialog)  Indices=2,3  OutputSizes=1,1
  Selector1 : Selector  NumberOfDimensions=2  InputPortWidth=3  IndexOptions=Index vector (dialog),Index vector (dialog)  Indices=3,2  OutputSizes=1,1
  Selector2 : Selector  NumberOfDimensions=2  InputPortWidth=3  IndexOptions=Index vector (dialog),Index vector (dialog)  Indices=3,1  OutputSizes=1,1
  Selector3 : Selector  NumberOfDimensions=2  InputPortWidth=3  IndexOptions=Index vector (dialog),Index vector (dialog)  Indices=1,3  OutputSizes=1,1
  Selector4 : Selector  NumberOfDimensions=2  InputPortWidth=3  IndexOptions=Index vector (dialog),Index vector (dialog)  Indices=1,2  OutputSizes=1,1
  Selector6 : Selector  NumberOfDimensions=2  InputPortWidth=3  IndexOptions=Index vector (dialog),Index vector (dialog)  Indices=2,1  OutputSizes=1,1
  Sum1 : Sum  Inputs=+-
  Sum2 : Sum
  Sum3 : Sum
  quaternion_1 : Outport
  wires:
  Selector2/1 -> Sum2/1  "A31"
  Divide2/1 -> Mux/2  "q2"
  Selector4/1 -> Sum3/1  "A12"
  Gain1/1 -> Divide/1
  Sum1/1 -> Gain1/1
  Gain2/1 -> Divide1/1
  Selector/1 -> Sum1/1  "A23"
  Divide1/1 -> Mux/3  "q3"
  Divide/1 -> Mux/4  "q4"
  q1/1 -> Divide2/2, Divide1/2, Divide/2, Mux/1
  Selector6/1 -> Sum3/2  "A21"
  "A_BN "/1 -> Selector/1, Selector1/1, Selector3/1, Selector4/1, Selector6/1, Selector2/1
  Sum3/1 -> Gain3/1
  Sum2/1 -> Gain2/1
  Gain3/1 -> Divide2/1
  Selector3/1 -> Sum2/2  "A13"
  Selector1/1 -> Sum1/2  "A32"
  Mux/1 -> quaternion_1/1

== system spacecraft_attitude_model/Slew & Pointing/Slew and Pointing/Subsystem1/If Action Subsystem3 ==
  q2 : Inport
  A_BN : Inport  Port=2
  Action Port : ActionPort  ActionPortLabel=elseif( u3>0 & u3<1)
  Divide : Product  Inputs=*/
  Divide1 : Product  Inputs=*/
  Divide2 : Product  Inputs=*/
  Gain1 : Gain  Gain=1/4
  Gain2 : Gain  Gain=1/4
  Gain3 : Gain  Gain=1/4
  Mux : Mux
  Selector : Selector  NumberOfDimensions=2  InputPortWidth=3  IndexOptions=Index vector (dialog),Index vector (dialog)  Indices=2,3  OutputSizes=1,1
  Selector1 : Selector  NumberOfDimensions=2  InputPortWidth=3  IndexOptions=Index vector (dialog),Index vector (dialog)  Indices=3,2  OutputSizes=1,1
  Selector2 : Selector  NumberOfDimensions=2  InputPortWidth=3  IndexOptions=Index vector (dialog),Index vector (dialog)  Indices=3,1  OutputSizes=1,1
  Selector3 : Selector  NumberOfDimensions=2  InputPortWidth=3  IndexOptions=Index vector (dialog),Index vector (dialog)  Indices=1,3  OutputSizes=1,1
  Selector4 : Selector  NumberOfDimensions=2  InputPortWidth=3  IndexOptions=Index vector (dialog),Index vector (dialog)  Indices=1,2  OutputSizes=1,1
  Selector6 : Selector  NumberOfDimensions=2  InputPortWidth=3  IndexOptions=Index vector (dialog),Index vector (dialog)  Indices=2,1  OutputSizes=1,1
  Sum1 : Sum
  Sum2 : Sum  Inputs=+-
  Sum3 : Sum
  quaternion_2 : Outport
  wires:
  Sum1/1 -> Gain1/1
  Gain1/1 -> Divide/1
  Selector6/1 -> Sum3/2  "A21"
  Selector/1 -> Sum1/1  "A23"
  Divide1/1 -> Mux/4  "q4"
  Selector2/1 -> Sum2/1  "A31"
  Gain2/1 -> Divide1/1
  Divide/1 -> Mux/3  "q3"
  Divide2/1 -> Mux/1  "q1"
  Selector1/1 -> Sum1/2  "A32"
  Selector3/1 -> Sum2/2  "A13"
  Gain3/1 -> Divide2/1
  Sum2/1 -> Gain2/1
  q2/1 -> Divide2/2, Divide1/2, Divide/2, Mux/2
  A_BN/1 -> Selector/1, Selector1/1, Selector3/1, Selector4/1, Selector6/1, Selector2/1
  Selector4/1 -> Sum3/1  "A12"
  Sum3/1 -> Gain3/1
  Mux/1 -> quaternion_2/1

== system spacecraft_attitude_model/Slew & Pointing/Slew and Pointing/Subsystem1/If Action Subsystem4 ==
  q3 : Inport
  "A_BN " : Inport  Port=2
  Action Port : ActionPort  ActionPortLabel=elseif( u4>0 & u4<1)
  Divide : Product  Inputs=*/
  Divide1 : Product  Inputs=*/
  Divide2 : Product  Inputs=*/
  Gain1 : Gain  Gain=1/4
  Gain2 : Gain  Gain=1/4
  Gain3 : Gain  Gain=1/4
  Mux : Mux
  Selector : Selector  NumberOfDimensions=2  InputPortWidth=3  IndexOptions=Index vector (dialog),Index vector (dialog)  Indices=2,3  OutputSizes=1,1
  Selector1 : Selector  NumberOfDimensions=2  InputPortWidth=3  IndexOptions=Index vector (dialog),Index vector (dialog)  Indices=3,2  OutputSizes=1,1
  Selector2 : Selector  NumberOfDimensions=2  InputPortWidth=3  IndexOptions=Index vector (dialog),Index vector (dialog)  Indices=3,1  OutputSizes=1,1
  Selector3 : Selector  NumberOfDimensions=2  InputPortWidth=3  IndexOptions=Index vector (dialog),Index vector (dialog)  Indices=1,3  OutputSizes=1,1
  Selector4 : Selector  NumberOfDimensions=2  InputPortWidth=3  IndexOptions=Index vector (dialog),Index vector (dialog)  Indices=1,2  OutputSizes=1,1
  Selector6 : Selector  NumberOfDimensions=2  InputPortWidth=3  IndexOptions=Index vector (dialog),Index vector (dialog)  Indices=2,1  OutputSizes=1,1
  Sum1 : Sum
  Sum2 : Sum
  Sum3 : Sum  Inputs=+-
  quaternion_3 : Outport
  wires:
  Sum3/1 -> Gain3/1
  Selector4/1 -> Sum3/1  "A12"
  Selector3/1 -> Sum2/2  "A13"
  Sum2/1 -> Gain2/1
  Gain3/1 -> Divide2/1
  Selector1/1 -> Sum1/2  "A32"
  Divide2/1 -> Mux/4  "q4"
  Gain2/1 -> Divide1/1
  Selector2/1 -> Sum2/1  "A31"
  Divide1/1 -> Mux/1  "q1"
  Gain1/1 -> Divide/1
  Selector/1 -> Sum1/1  "A23"
  Selector6/1 -> Sum3/2  "A21"
  Sum1/1 -> Gain1/1
  Divide/1 -> Mux/2  "q2"
  q3/1 -> Mux/3, Divide2/2, Divide1/2, Divide/2
  "A_BN "/1 -> Selector/1, Selector1/1, Selector3/1, Selector4/1, Selector6/1, Selector2/1
  Mux/1 -> quaternion_3/1

== system spacecraft_attitude_model/Slew & Pointing/Slew and Pointing/Subsystem1/If Action Subsystem5 ==
  In1 : Inport
  Action Port : ActionPort  ActionPortLabel=else
  Demux : Demux
  Demux1 : Demux
  Product{,1..4} (5 alike) : Product
  Sign : Signum
  Sum : Sum  Inputs=++++
  Zero-Order Hold : ZeroOrderHold  SampleTime=-1
  q : Outport
  wires:
  Demux/3 -> Product1/1
  Product4/1 -> q/1
  Sum/1 -> Sign/1  "J"
  Demux1/2 -> Product2/2
  Zero-Order Hold/1 -> Demux1/1
  Product/1 -> Sum/4
  Demux/4 -> Product/1
  Product1/1 -> Sum/3
  Demux1/4 -> Product/2
  Sign/1 -> Product4/1
  Demux/1 -> Product3/1
  Demux1/1 -> Product3/2
  Product2/1 -> Sum/2
  Product3/1 -> Sum/1
  Demux/2 -> Product2/1
  Demux1/3 -> Product1/2
  In1/1 -> Product4/2, Demux/1, Zero-Order Hold/1

== system spacecraft_attitude_model/Slew & Pointing/Slew and Pointing/Subsystem1/Ortonormalization ==
  A_LN : Inport
  Gain : Gain  Gain=3/2
  Gain1 : Gain  Gain=1/2
  Product : Product  Multiplication=Matrix(*)
  Product1 : Product  Multiplication=Matrix(*)
  Sum : Sum  Inputs=|+-
  Transpose : Math  Operator=transpose
  Out1 : Outport
  wires:
  A_LN/1 -> Product1/2, Product/2, Transpose/1, Gain/1
  Gain/1 -> Sum/1
  Gain1/1 -> Sum/2
  Sum/1 -> Out1/1
  Transpose/1 -> Product/1
  Product/1 -> Product1/1
  Product1/1 -> Gain1/1

== system spacecraft_attitude_model/Slew & Pointing/Slew and Pointing/Subsystem1/Subsystem ==
  A_BN : Inport
  Constant : Constant
  Gain : Gain  Gain=1/2
  Selector5 : Selector  NumberOfDimensions=2  InputPortWidth=3  IndexOptions=Index vector (dialog),Index vector (dialog)  Indices=1,1  OutputSizes=1,1
  Selector7 : Selector  NumberOfDimensions=2  InputPortWidth=3  IndexOptions=Index vector (dialog),Index vector (dialog)  Indices=2,2  OutputSizes=1,1
  Selector8 : Selector  NumberOfDimensions=2  InputPortWidth=3  IndexOptions=Index vector (dialog),Index vector (dialog)  Indices=3,3  OutputSizes=1,1
  Sqrt : Sqrt
  Sum : Sum  Inputs=++++
  q4 : Outport
  wires:
  A_BN/1 -> Selector5/1, Selector8/1, Selector7/1
  Selector5/1 -> Sum/1  "A11"
  Sqrt/1 -> Gain/1
  Selector8/1 -> Sum/3  "A33"
  Sum/1 -> Sqrt/1
  Selector7/1 -> Sum/2  "A22"
  Constant/1 -> Sum/4
  Gain/1 -> q4/1  "q4"

== system spacecraft_attitude_model/Slew & Pointing/Slew and Pointing/Subsystem1/Subsystem1 ==
  A_BN : Inport
  Constant : Constant
  Gain : Gain  Gain=1/2
  Selector5 : Selector  NumberOfDimensions=2  InputPortWidth=3  IndexOptions=Index vector (dialog),Index vector (dialog)  Indices=1,1  OutputSizes=1,1
  Selector7 : Selector  NumberOfDimensions=2  InputPortWidth=3  IndexOptions=Index vector (dialog),Index vector (dialog)  Indices=2,2  OutputSizes=1,1
  Selector8 : Selector  NumberOfDimensions=2  InputPortWidth=3  IndexOptions=Index vector (dialog),Index vector (dialog)  Indices=3,3  OutputSizes=1,1
  Sqrt : Sqrt
  Sum : Sum  Inputs=+--+
  q1 : Outport
  wires:
  Selector7/1 -> Sum/2  "A22"
  Selector5/1 -> Sum/1  "A11"
  A_BN/1 -> Selector5/1, Selector7/1, Selector8/1
  Selector8/1 -> Sum/3  "A33"
  Sum/1 -> Sqrt/1
  Constant/1 -> Sum/4
  Gain/1 -> q1/1  "q1"
  Sqrt/1 -> Gain/1

== system spacecraft_attitude_model/Slew & Pointing/Slew and Pointing/Subsystem1/Subsystem2 ==
  A_BN : Inport
  Constant : Constant
  Gain : Gain  Gain=1/2
  Selector5 : Selector  NumberOfDimensions=2  InputPortWidth=3  IndexOptions=Index vector (dialog),Index vector (dialog)  Indices=1,1  OutputSizes=1,1
  Selector7 : Selector  NumberOfDimensions=2  InputPortWidth=3  IndexOptions=Index vector (dialog),Index vector (dialog)  Indices=2,2  OutputSizes=1,1
  Selector8 : Selector  NumberOfDimensions=2  InputPortWidth=3  IndexOptions=Index vector (dialog),Index vector (dialog)  Indices=3,3  OutputSizes=1,1
  Sqrt : Sqrt
  Sum : Sum  Inputs=-+-+
  q2 : Outport
  wires:
  Selector5/1 -> Sum/1  "A11"
  Sqrt/1 -> Gain/1
  Constant/1 -> Sum/4
  Gain/1 -> q2/1  "q2"
  Sum/1 -> Sqrt/1
  Selector8/1 -> Sum/3  "A33"
  Selector7/1 -> Sum/2  "A22"
  A_BN/1 -> Selector5/1, Selector8/1, Selector7/1

== system spacecraft_attitude_model/Slew & Pointing/Slew and Pointing/Subsystem1/Subsystem3 ==
  A_BN : Inport
  Constant : Constant
  Gain : Gain  Gain=1/2
  Selector5 : Selector  NumberOfDimensions=2  InputPortWidth=3  IndexOptions=Index vector (dialog),Index vector (dialog)  Indices=1,1  OutputSizes=1,1
  Selector7 : Selector  NumberOfDimensions=2  InputPortWidth=3  IndexOptions=Index vector (dialog),Index vector (dialog)  Indices=2,2  OutputSizes=1,1
  Selector8 : Selector  NumberOfDimensions=2  InputPortWidth=3  IndexOptions=Index vector (dialog),Index vector (dialog)  Indices=3,3  OutputSizes=1,1
  Sqrt : Sqrt
  Sum : Sum  Inputs=--++
  q3 : Outport
  wires:
  Selector7/1 -> Sum/2  "A22"
  Gain/1 -> q3/1  "q3"
  Sqrt/1 -> Gain/1
  Constant/1 -> Sum/4
  A_BN/1 -> Selector5/1, Selector8/1, Selector7/1
  Selector8/1 -> Sum/3  "A33"
  Selector5/1 -> Sum/1  "A11"
  Sum/1 -> Sqrt/1

== system spacecraft_attitude_model/Slew & Pointing/Slew and Pointing/Subsystem2/If Action Subsystem1 ==
  Input : Inport
  Action Port : ActionPort  ActionPortLabel=if(u1==0)
  q : Outport
  wires:
  Input/1 -> q/1

== system spacecraft_attitude_model/Slew & Pointing/Slew and Pointing/Subsystem2/If Action Subsystem5 ==
  In1 : Inport
  Action Port : ActionPort  ActionPortLabel=else
  Complex to Real-Imag : ComplexToRealImag  Commented=on
  Dot Product : DotProduct  OutDataTypeStr=Inherit: Inherit via internal rule
  Memory : Memory  Commented=on
  Product4 : Product
  Scope1 : Scope
  Sign : Signum
  Unit Delay : UnitDelay  InitialCondition=[0 0 0 1]'  SampleTime=-1  HasFrameUpgradeWarning=on
  q_ : Outport
  wires:
  Dot Product/1 -> Scope1/1, Sign/1  "J"
  Sign/1 -> Product4/1
  In1/1 -> Dot Product/1, Product4/2
  Product4/1 -> Unit Delay/1, q_/1
  Unit Delay/1 -> Dot Product/2

== system spacecraft_attitude_model/Slew & Pointing/Subsystem/Magnetic coils/Norm1 ==
  b : Inport
  Demux : Demux  Outputs=3
  Sqrt : Sqrt
  Square : Math  Operator=square
  Square1 : Math  Operator=square
  Square2 : Math  Operator=square
  Sum : Sum  Inputs=|+++
  b_norm : Outport
  wires:
  Demux/3 -> Square2/1
  b/1 -> Demux/1
  Demux/1 -> Square/1
  Demux/2 -> Square1/1
  Square/1 -> Sum/1
  Square1/1 -> Sum/2
  Square2/1 -> Sum/3
  Sum/1 -> Sqrt/1
  Sqrt/1 -> b_norm/1

== system spacecraft_attitude_model/Slew & Pointing/Subsystem/Magnetic coils/Subsystem ==
  T_x : Inport
  b_x : Inport  Port=2
  b_norm^2 : Inport  Port=3
  Divide2 : Product  Inputs=*/
  Product : Product
  Product1 : Product
  Saturation2 : Saturate  UpperLimit=T_coil_max  LowerLimit=-T_coil_max
  Saturation3 : Saturate  UpperLimit=D_max  LowerLimit=-D_max
  Scope2 : Scope
  Scope3 : Scope
  T_coil_x : Outport
  wires:
  Saturation3/1 -> Product1/1
  Divide2/1 -> Scope3/1, Saturation3/1
  Product/1 -> Divide2/1
  Product1/1 -> Saturation2/1  "T_coils_x"
  b_norm^2/1 -> Divide2/2
  b_x/1 -> Product1/2, Product/2
  T_x/1 -> Product/1
  Saturation2/1 -> Scope2/1, T_coil_x/1

== system spacecraft_attitude_model/Slew & Pointing/Subsystem/Magnetic coils/Subsystem1 ==
  T_y : Inport
  b_y : Inport  Port=2
  b_norm^2 : Inport  Port=3
  Divide2 : Product  Inputs=*/
  Product : Product
  Product1 : Product
  Saturation2 : Saturate  UpperLimit=T_coil_max  LowerLimit=-T_coil_max
  Saturation3 : Saturate  UpperLimit=D_max  LowerLimit=-D_max
  Scope2 : Scope
  Scope3 : Scope
  T_coil_y : Outport
  wires:
  Saturation3/1 -> Product1/1
  Divide2/1 -> Scope3/1, Saturation3/1
  Product/1 -> Divide2/1
  Product1/1 -> Saturation2/1
  b_norm^2/1 -> Divide2/2
  b_y/1 -> Product1/2, Product/2
  T_y/1 -> Product/1
  Saturation2/1 -> Scope2/1, T_coil_y/1
